simulink model "MR_simulink"  (R2025b)
settings: Solver=VariableStepAuto  StartTime=0.0  StopTime=10.0  RelTol=1e-3
libraries: fl_lib x2
settings Model: Creator=leona  LastModifiedBy=leona

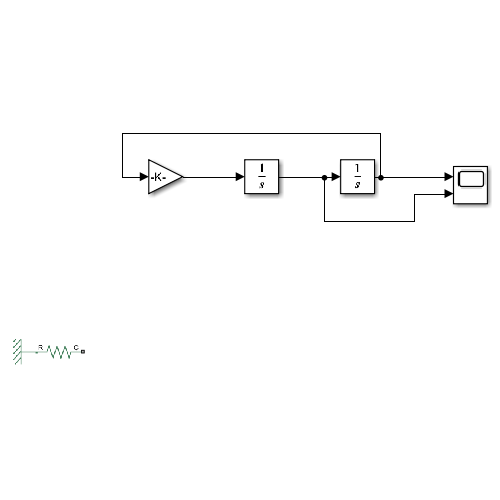
[thumbnail: Simulink's stored preview of the top-level diagram]
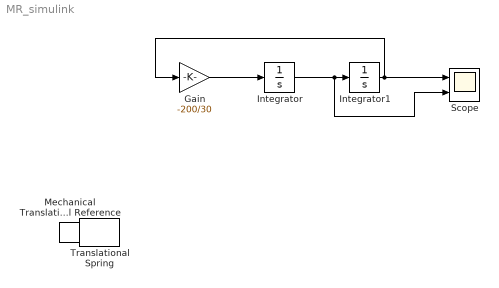
== system MR_simulink ==
  Gain : Gain  Gain=-200/30
  Integrator : Integrator  InitialCondition=2
  Integrator1 : Integrator
  Mechanical Translational Reference : fl_lib/Mechanical/Translational Elements/Mechanical Translational Reference
  Scope : Scope  NumInputPorts=2
      settings: ActiveDisplayYMinimum=-2.4995493874118857  ActiveDisplayYMaximum=2.4999499319346539
  Translational Spring : fl_lib/Mechanical/Translational Elements/Translational Spring  spr_rate=1000 N/m  v_specify=off  v_priority=None  v=0 m/s  v_nominal_specify=off  v_nominal_value=1  v_nominal_unit=m/s  f_specify=off  f_priority=None  f=0 N  f_nominal_specify=off  f_nominal_value=1  f_nominal_unit=N  x_specify=off  x_priority=High  x=0 m  x_nominal_specify=off  x_nominal_value=1  x_nominal_unit=m
  wires:
  Integrator/1 -> Scope/2, Integrator1/1
  Integrator1/1 -> Gain/1, Scope/1
  Gain/1 -> Integrator/1
  connections:
  Mechanical Translational Reference/LConn1 -- Translational Spring/LConn1
